simulink model "modulator_demodulator"  (R2021b)
settings: Solver=VariableStepAuto  StartTime=0.0  StopTime=10.0  RelTol=1e-3
undefined symbols (not defined in the file): magnitude
libraries: dsparch4 x1
settings Model: Creator=Joshua  LastModifiedBy=Joshua

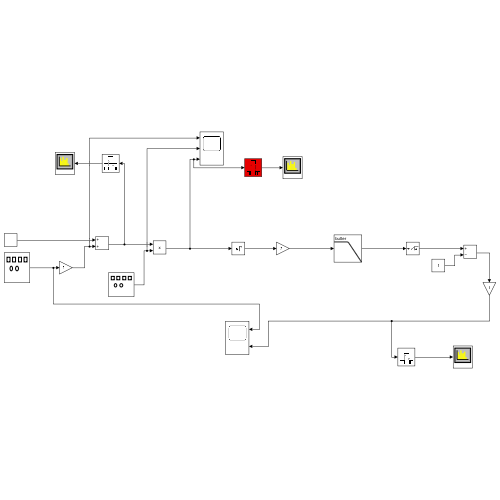
[thumbnail: Simulink's stored preview of the top-level diagram]
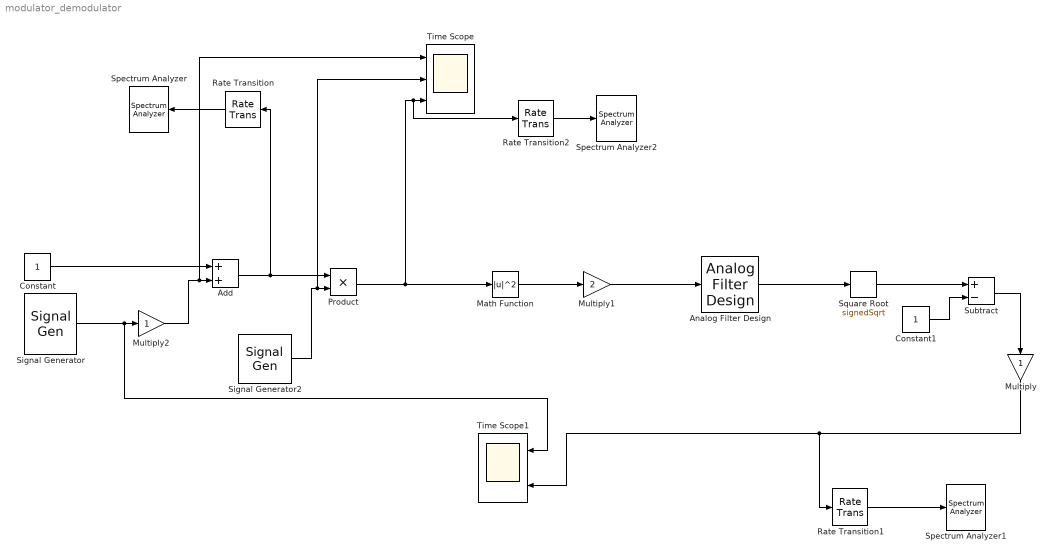
== system modulator_demodulator ==
  Add : Sum
  Analog Filter Design : dsparch4/Analog Filter Design  method=Butterworth  filttype=Lowpass  N=8  Wlo=30  Whi=80  Rp=2  Rs=40
  Constant : Constant
  Constant1 : Constant
  Math Function : Math  Operator=magnitude^2  SaturateOnIntegerOverflow=on
  Multiply : Gain
  Multiply1 : Gain  Gain=2
  Multiply2 : Gain
  Product : Product
  Rate Transition : RateTransition
  Rate Transition1 : RateTransition
  Rate Transition2 : RateTransition
  Signal Generator : SignalGenerator  Units=rad/sec
  Signal Generator2 : SignalGenerator  Units=rad/sec
  Spectrum Analyzer : SpectrumAnalyzer
  Spectrum Analyzer1 : SpectrumAnalyzer
  Spectrum Analyzer2 : SpectrumAnalyzer
  Square Root : Sqrt  Operator=signedSqrt  SaturateOnIntegerOverflow=on
  Subtract : Sum  Inputs=+-
  Time Scope : Scope  NumInputPorts=3
  Time Scope1 : Scope  NumInputPorts=2
  wires:
  Signal Generator2/1 -> Time Scope/2, Product/2
  Product/1 -> Math Function/1, Rate Transition2/1, Time Scope/3
  Math Function/1 -> Multiply1/1
  Multiply1/1 -> Analog Filter Design/1
  Analog Filter Design/1 -> Square Root/1
  Constant1/1 -> Subtract/2
  Square Root/1 -> Subtract/1
  Signal Generator/1 -> Time Scope1/1, Multiply2/1
  Multiply2/1 -> Time Scope/1, Add/2
  Add/1 -> Rate Transition/1, Product/1
  Constant/1 -> Add/1
  Rate Transition/1 -> Spectrum Analyzer/1
  Subtract/1 -> Multiply/1
  Multiply/1 -> Rate Transition1/1, Time Scope1/2
  Rate Transition1/1 -> Spectrum Analyzer1/1
  Rate Transition2/1 -> Spectrum Analyzer2/1
